simulink model "impedanceWithTorque"  (R2019a)
settings: Solver=ode4  StartTime=0.0  StopTime=60  FixedStep=0.01  RelTol=1e-3
undefined symbols (not defined in the file or in its folder): KI
libraries: dspswit3 x3
settings Model: Creator=JanAriel  LastModifiedBy=sensei

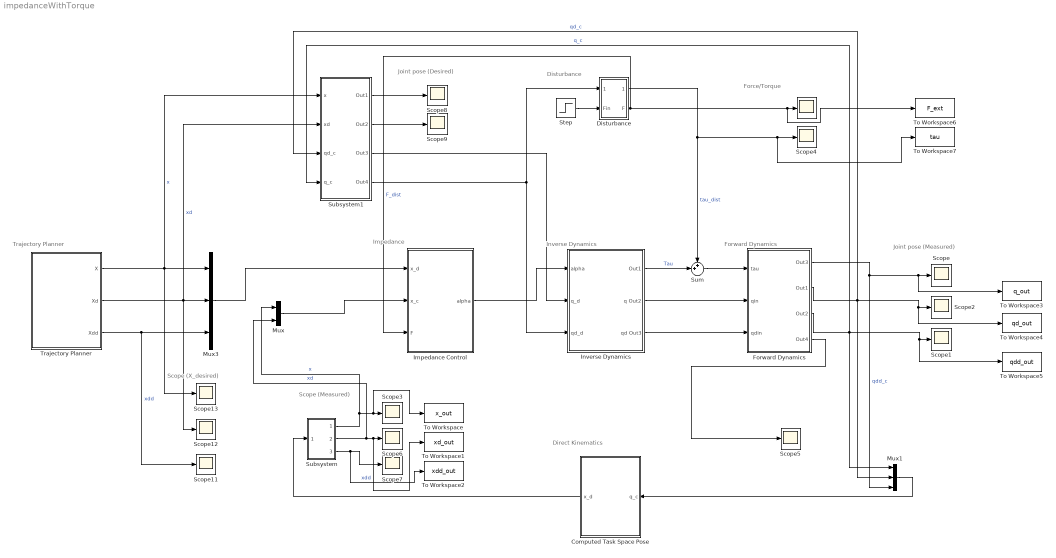
== system impedanceWithTorque ==
  note: Disturbance
  note: Scope (X_desired)
  note: Joint pose (Measured)
  note: Direct Kinematics
  note: Scope (Measured)
  note: Force/Torque
  note: Forward Dynamics
  note: Inverse Dynamics
  note: Impedance
  note: Joint pose (Desired)
  note: Trajectory Planner
  " " : Scope
  Computed Task Space Pose : Subsystem
  Disturbance : Subsystem
  Forward Dynamics : Subsystem
  Impedance Control : Subsystem
  Inverse Dynamics : Subsystem
  Mux : Mux  Inputs=2
  Mux1 : Mux  Inputs=3
  Mux3 : Mux  Inputs=3
  Scope{,1..9,11..13} (13 alike) : Scope
  Step : Step  Time=15  After=[1;1;0]  SampleTime=0  VectorParams1D=off
  Subsystem : Subsystem
  Subsystem1 : Subsystem
  Sum : Sum  Inputs=++|
  To Workspace : ToWorkspace  VariableName=x_out  SaveFormat=Structure With Time  SampleTime=-1
  To Workspace1 : ToWorkspace  VariableName=xd_out  SaveFormat=Structure With Time  SampleTime=-1
  To Workspace2 : ToWorkspace  VariableName=xdd_out  SaveFormat=Structure With Time  SampleTime=-1
  To Workspace3 : ToWorkspace  VariableName=q_out  SaveFormat=Structure With Time  SampleTime=-1
  To Workspace4 : ToWorkspace  VariableName=qd_out  SaveFormat=Structure With Time  SampleTime=-1
  To Workspace5 : ToWorkspace  VariableName=qdd_out  SaveFormat=Structure With Time  SampleTime=-1
  To Workspace6 : ToWorkspace  VariableName=F_ext  SaveFormat=Structure With Time  SampleTime=-1
  To Workspace7 : ToWorkspace  VariableName=tau  SaveFormat=Structure With Time  SampleTime=-1
  Trajectory Planner : Subsystem
  wires:
  Inverse Dynamics/3(qd Out3) -> Forward Dynamics/3(qdin)
  Trajectory Planner/3(Xdd) -> Scope11/1, Mux3/3  "xdd"
  Subsystem/1(Out1) -> To Workspace/1, Scope3/1, Mux/1  "x"
  Subsystem/3(Out3) -> To Workspace2/1, Scope7/1  "xdd"
  Subsystem/2(Out2) -> Mux/2, To Workspace1/1, Scope6/1  "xd"
  Forward Dynamics/2(Out1) -> Subsystem1/3(qd_c), Mux1/2, To Workspace4/1, Scope2/1  "qd_c"
  Forward Dynamics/1(Out3) -> To Workspace3/1, Scope/1, Mux1/3  "qdd_c"
  Inverse Dynamics/1(Out1) -> Sum/2  "Tau"
  Inverse Dynamics/2(q Out2) -> Forward Dynamics/2(qin)
  Mux1/1 -> Computed Task Space Pose/1(q_c)
  Subsystem1/4(Out4) -> Disturbance/1(In1), Inverse Dynamics/3(qd_d)
  Subsystem1/3(Out3) -> Inverse Dynamics/2(q_d)
  Subsystem1/1(Out1) -> Scope8/1
  Trajectory Planner/2(Xd) -> Scope12/1, Subsystem1/2(xd), Mux3/2  "xd"
  Mux3/1 -> Impedance Control/1(x_d)
  Trajectory Planner/1(X) -> Scope13/1, Subsystem1/1(x), Mux3/1  "x"
  Impedance Control/1(alpha) -> Inverse Dynamics/1(alpha)
  Computed Task Space Pose/1(x_d) -> Subsystem/1(In1)
  Mux/1 -> Impedance Control/2(x_c)
  Subsystem1/2(Out2) -> Scope9/1
  Forward Dynamics/3(Out2) -> To Workspace5/1, Scope1/1, Mux1/1, Subsystem1/4(q_c)  "q_c"
  Sum/1 -> Forward Dynamics/1(tau)
  Disturbance/1(Tau) -> To Workspace7/1, Scope4/1, Sum/1  "tau_dist"
  Disturbance/2(F) -> Impedance Control/3(F), To Workspace6/1, " "/1  "F_dist"
  Step/1 -> Disturbance/2(Fin)
  Forward Dynamics/4(Out4) -> Scope5/1

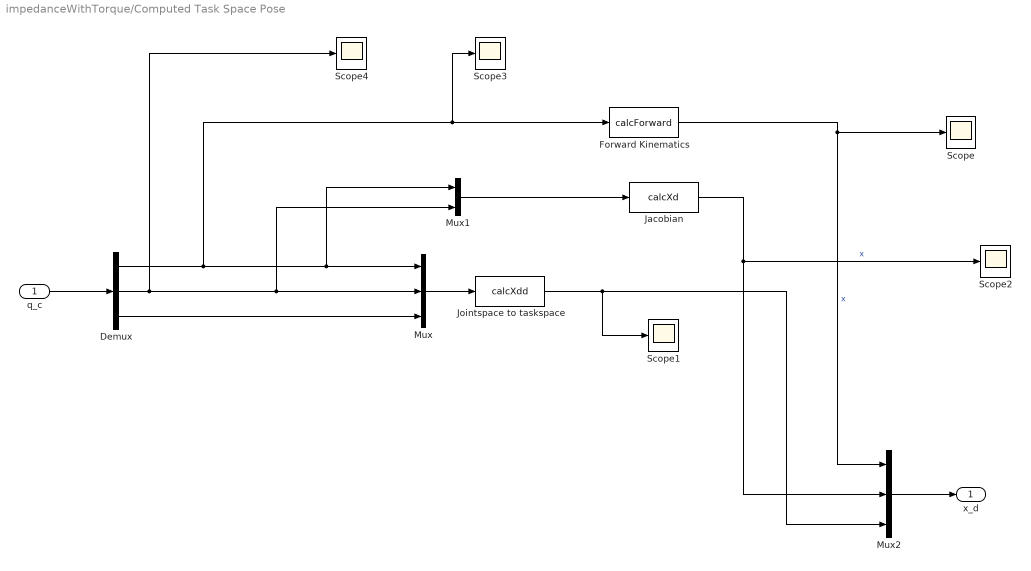
== system impedanceWithTorque/Computed Task Space Pose ==
  q_c : Inport
  Demux : Demux  Outputs=3
  Forward Kinematics : MATLABFcn  MATLABFcn=calcForward  Output1D=off
  Jacobian : MATLABFcn  MATLABFcn=calcXd  Output1D=off
  Jointspace to taskspace : MATLABFcn  MATLABFcn=calcXdd  Output1D=off
  Mux : Mux  Inputs=3
  Mux1 : Mux  Inputs=2
  Mux2 : Mux  Inputs=3
  Scope{,1..4} (5 alike) : Scope
  x_d : Outport
  wires:
  q_c/1 -> Demux/1
  Mux/1 -> Jointspace to taskspace/1
  Demux/2 -> Scope4/1, Mux/2, Mux1/2
  Forward Kinematics/1 -> Mux2/1, Scope/1  "x"
  Demux/1 -> Scope3/1, Forward Kinematics/1, Mux/1, Mux1/1
  Mux1/1 -> Jacobian/1
  Demux/3 -> Mux/3
  Jointspace to taskspace/1 -> Scope1/1, Mux2/3
  Mux2/1 -> x_d/1
  Jacobian/1 -> Scope2/1, Mux2/2  "x"

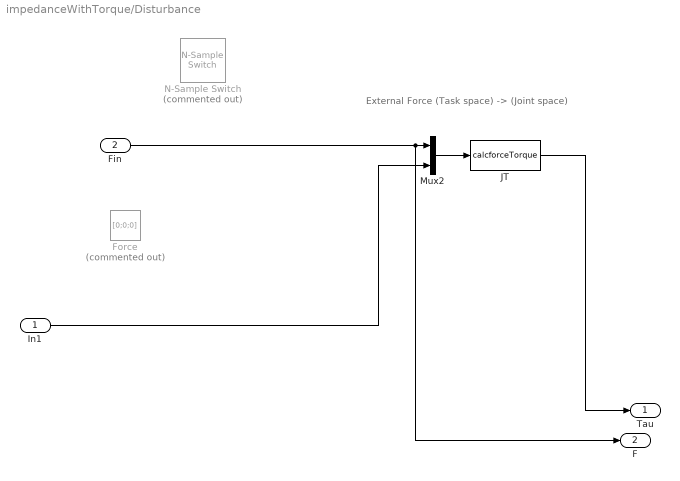
== system impedanceWithTorque/Disturbance ==
  note: External Force (Task space) -> (Joint space)
  In1 : Inport
  Fin : Inport  Port=2
  Force : Constant  Commented=on  Value=[0;0;0]
  JT : MATLABFcn  MATLABFcn=calcforceTorque  Output1D=off
  Mux2 : Mux  Inputs=2
  N-Sample Switch : dspswit3/N-Sample Switch  Commented=on  N=6000  reset=off  TriggerType=Rising edge  Ts=0.01
      settings: SourceProductName=DSP System Toolbox  SourceProductBaseCode=DS
  Tau : Outport
  F : Outport  Port=2
  wires:
  In1/1 -> Mux2/2
  JT/1 -> Tau/1
  Mux2/1 -> JT/1
  Fin/1 -> F/1, Mux2/1

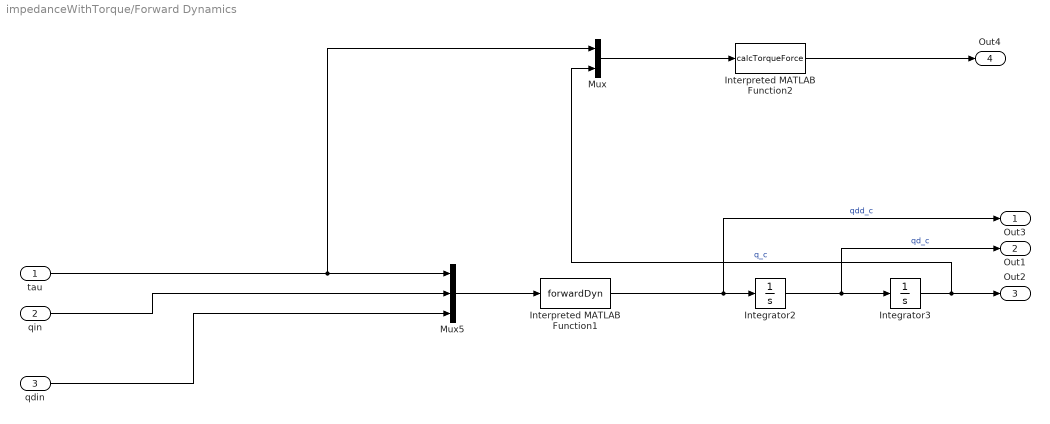
== system impedanceWithTorque/Forward Dynamics ==
  tau : Inport
  qin : Inport  Port=2
  qdin : Inport  Port=3
  Integrator2 : Integrator
  Integrator3 : Integrator
  Interpreted MATLAB Function1 : MATLABFcn  MATLABFcn=forwardDyn  Output1D=off
  Interpreted MATLAB Function2 : MATLABFcn  MATLABFcn=calcTorqueForce  Output1D=off
  Mux : Mux  Inputs=2
  Mux5 : Mux  Inputs=3
  Out3 : Outport
  Out1 : Outport  Port=2
  Out2 : Outport  Port=3
  Out4 : Outport  Port=4
  wires:
  Integrator2/1 -> Integrator3/1, Out1/1  "qd_c"
  Integrator3/1 -> Mux/2, Out2/1  "q_c"
  Interpreted MATLAB Function1/1 -> Out3/1, Integrator2/1  "qdd_c"
  tau/1 -> Mux/1, Mux5/1
  qin/1 -> Mux5/2
  qdin/1 -> Mux5/3
  Mux5/1 -> Interpreted MATLAB Function1/1
  Interpreted MATLAB Function2/1 -> Out4/1
  Mux/1 -> Interpreted MATLAB Function2/1

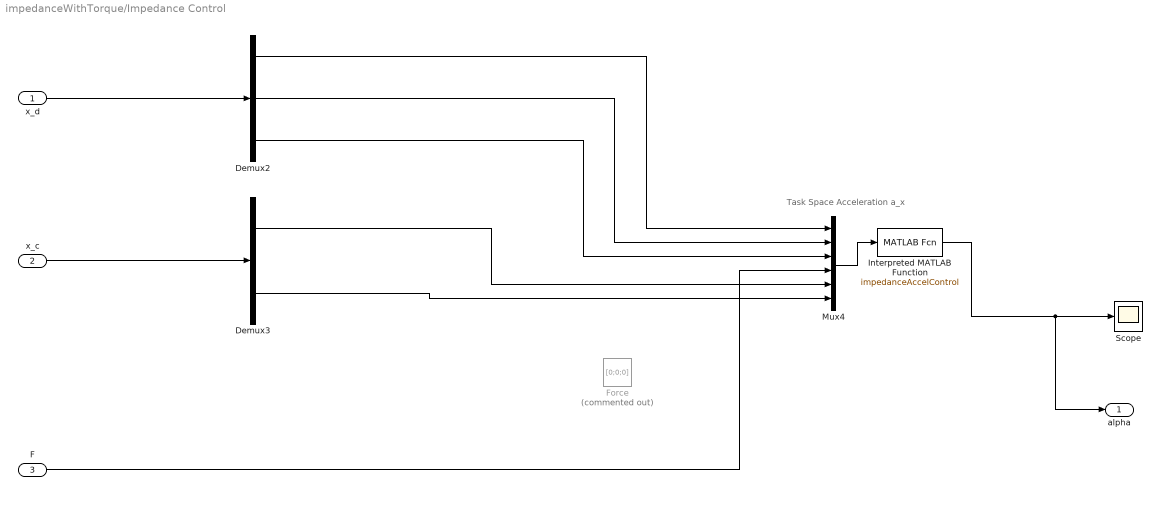
== system impedanceWithTorque/Impedance Control ==
  note: Task Space Acceleration a_x
  x_d : Inport
  x_c : Inport  Port=2
  F : Inport  Port=3
  Demux2 : Demux  Outputs=3
  Demux3 : Demux  Outputs=2
  Force : Constant  Commented=on  Value=[0;0;0]
  Interpreted MATLAB Function : MATLABFcn  MATLABFcn=impedanceAccelControl  Output1D=off
  Mux4 : Mux  Inputs=6
  Scope : Scope
  alpha : Outport
  wires:
  Demux2/2 -> Mux4/2
  Demux2/1 -> Mux4/1
  Demux2/3 -> Mux4/3
  Mux4/1 -> Interpreted MATLAB Function/1
  Interpreted MATLAB Function/1 -> alpha/1, Scope/1
  x_d/1 -> Demux2/1
  Demux3/1 -> Mux4/5
  Demux3/2 -> Mux4/6
  x_c/1 -> Demux3/1
  F/1 -> Mux4/4

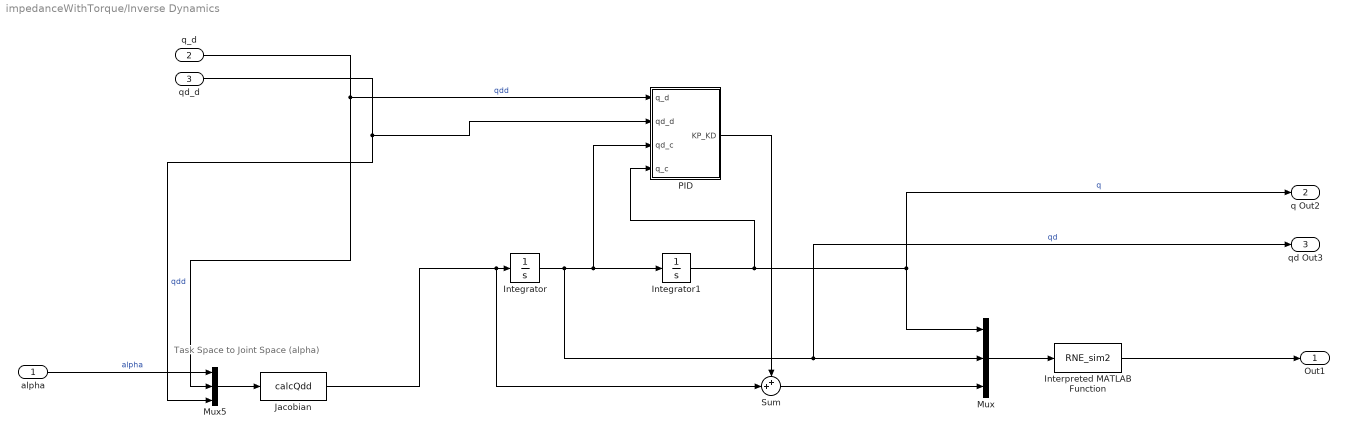
== system impedanceWithTorque/Inverse Dynamics ==
  note: Task Space to Joint Space (alpha)
  alpha : Inport
  q_d : Inport  Port=2
  qd_d : Inport  Port=3
  Integrator : Integrator
  Integrator1 : Integrator
  Interpreted MATLAB Function : MATLABFcn  MATLABFcn=RNE_sim2  Output1D=off
  Jacobian : MATLABFcn  MATLABFcn=calcQdd  Output1D=off
  Mux : Mux  Inputs=3
  Mux5 : Mux  Inputs=3
  PID : Subsystem
  Sum : Sum  Inputs=++|
  Out1 : Outport
  q Out2 : Outport  Port=2
  qd Out3 : Outport  Port=3
  wires:
  Mux/1 -> Interpreted MATLAB Function/1
  Interpreted MATLAB Function/1 -> Out1/1
  Integrator/1 -> PID/3(qd_c), Integrator1/1, Mux/2, qd Out3/1  "qd"
  Integrator1/1 -> PID/4(q_c), q Out2/1, Mux/1  "q"
  qd_d/1 -> Mux5/3, PID/2(qd_d)  "qdd"
  q_d/1 -> Mux5/2, PID/1(q_d)  "qdd"
  PID/1(KP_KD) -> Sum/1
  Sum/1 -> Mux/3
  Mux5/1 -> Jacobian/1
  alpha/1 -> Mux5/1  "alpha"
  Jacobian/1 -> Sum/2, Integrator/1

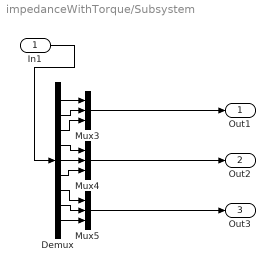
== system impedanceWithTorque/Subsystem ==
  In1 : Inport
  Demux : Demux  Outputs=9
  Mux3 : Mux  Inputs=3
  Mux4 : Mux  Inputs=3
  Mux5 : Mux  Inputs=3
  Out1 : Outport
  Out2 : Outport  Port=2
  Out3 : Outport  Port=3
  wires:
  Demux/8 -> Mux5/2
  Demux/7 -> Mux5/1
  Demux/1 -> Mux3/1
  Demux/3 -> Mux3/3
  Demux/9 -> Mux5/3
  Demux/6 -> Mux4/3
  Demux/5 -> Mux4/2
  Demux/4 -> Mux4/1
  Demux/2 -> Mux3/2
  Mux5/1 -> Out3/1
  In1/1 -> Demux/1
  Mux4/1 -> Out2/1
  Mux3/1 -> Out1/1

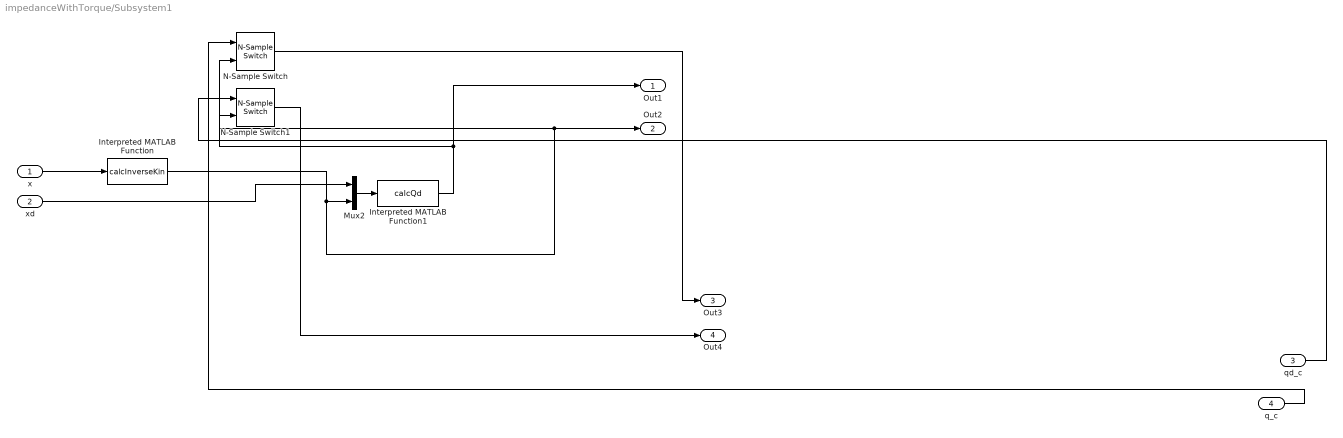
== system impedanceWithTorque/Subsystem1 ==
  x : Inport
  xd : Inport  Port=2
  qd_c : Inport  Port=3
  q_c : Inport  Port=4
  Interpreted MATLAB Function : MATLABFcn  MATLABFcn=calcInverseKin  Output1D=off
  Interpreted MATLAB Function1 : MATLABFcn  MATLABFcn=calcQd  Output1D=off
  Mux2 : Mux  Inputs=2
  N-Sample Switch : dspswit3/N-Sample Switch  N=1  reset=off  TriggerType=Rising edge  Ts=0.01
      settings: SourceProductName=DSP System Toolbox  SourceProductBaseCode=DS
  N-Sample Switch1 : dspswit3/N-Sample Switch  N=1  reset=off  TriggerType=Rising edge  Ts=0.01
      settings: SourceProductName=DSP System Toolbox  SourceProductBaseCode=DS
  Out1 : Outport
  Out2 : Outport  Port=2
  Out3 : Outport  Port=3
  Out4 : Outport  Port=4
  wires:
  xd/1 -> Mux2/1
  Interpreted MATLAB Function1/1 -> Out1/1, N-Sample Switch1/2
  N-Sample Switch1/1 -> Out4/1
  Interpreted MATLAB Function/1 -> Out2/1, N-Sample Switch/2, Mux2/2
  Mux2/1 -> Interpreted MATLAB Function1/1
  qd_c/1 -> N-Sample Switch1/1
  N-Sample Switch/1 -> Out3/1
  x/1 -> Interpreted MATLAB Function/1
  q_c/1 -> N-Sample Switch/1

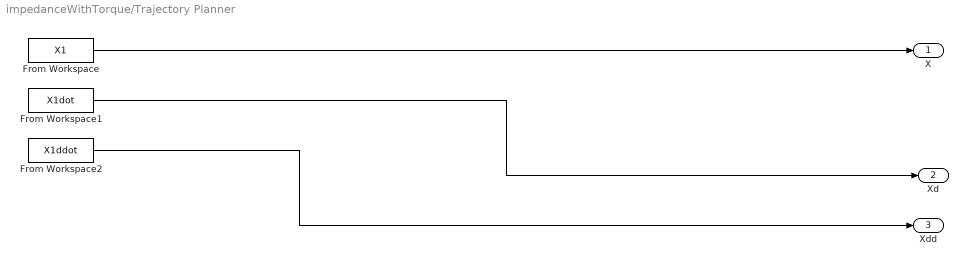
== system impedanceWithTorque/Trajectory Planner ==
  From Workspace : FromWorkspace  VariableName=X1  SampleTime=0
  From Workspace1 : FromWorkspace  VariableName=X1dot  SampleTime=0
  From Workspace2 : FromWorkspace  VariableName=X1ddot  SampleTime=0
  X : Outport
  Xd : Outport  Port=2
  Xdd : Outport  Port=3
  wires:
  From Workspace/1 -> X/1
  From Workspace1/1 -> Xd/1
  From Workspace2/1 -> Xdd/1

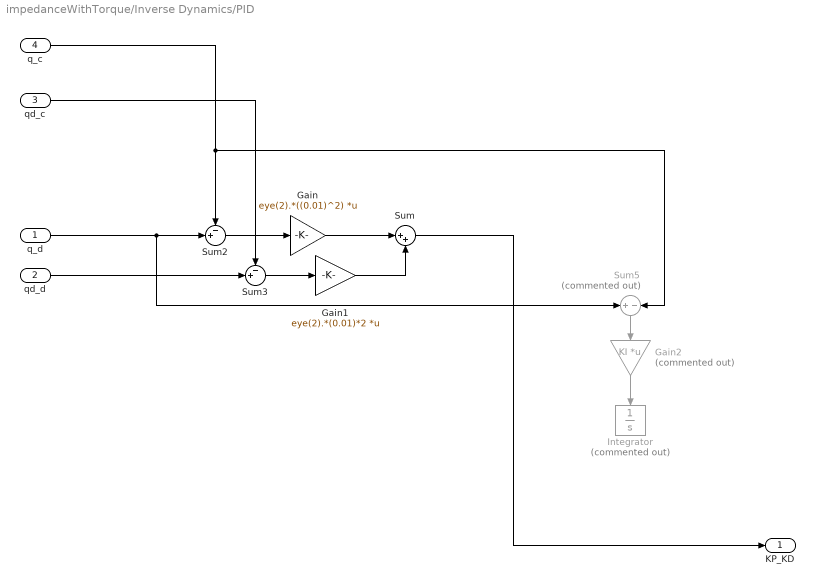
== system impedanceWithTorque/Inverse Dynamics/PID ==
  q_d : Inport
  qd_d : Inport  Port=2
  qd_c : Inport  Port=3
  q_c : Inport  Port=4
  Gain : Gain  Gain=eye(2).*((0.01)^2)  Multiplication=Matrix(K*u) (u vector)
  Gain1 : Gain  Gain=eye(2).*(0.01)*2  Multiplication=Matrix(K*u) (u vector)
  Gain2 : Gain  Commented=on  Gain=KI  Multiplication=Matrix(K*u) (u vector)
  Integrator : Integrator  Commented=on
  Sum : Sum  Inputs=|++
  Sum2 : Sum  Inputs=-+|
  Sum3 : Sum  Inputs=-+|
  Sum5 : Sum  Commented=on  Inputs=+-
  KP_KD : Outport
  wires:
  q_c/1 -> Sum5/2, Sum2/1
  Sum5/1 -> Gain2/1
  q_d/1 -> Sum2/2, Sum5/1
  Sum2/1 -> Gain/1
  Sum3/1 -> Gain1/1
  Gain2/1 -> Integrator/1
  Gain1/1 -> Sum/2
  Gain/1 -> Sum/1
  qd_c/1 -> Sum3/1
  Sum/1 -> KP_KD/1
  qd_d/1 -> Sum3/2
